simulink model "Scaler"  (Simulink 7.0)
settings: Solver=ode45  StartTime=0.0  StopTime=10.0  RelTol=1e-3
settings Model: Creator=volgy  LastModifiedBy=volgy

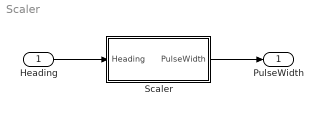
== system Scaler ==
  Heading : Inport  OutDataType=sfix(16)  OutScaling=2^0
  Scaler : Subsystem
  PulseWidth : Outport  OutDataType=sfix(16)  OutScaling=2^0
  wires:
  Heading/1 -> Scaler/1(Heading)
  Scaler/1(PulseWidth) -> PulseWidth/1

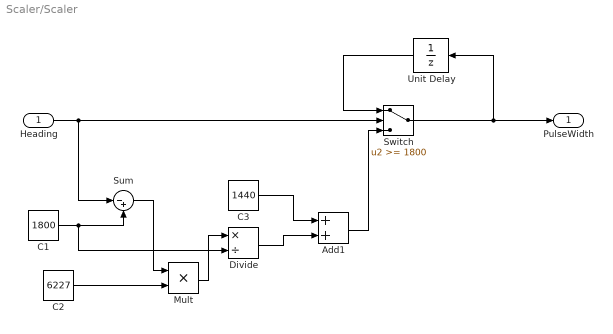
== system Scaler/Scaler ==
  Heading : Inport  OutDataType=sfix(16)  OutScaling=2^0
  Add1 : Sum  OutDataType=sfix(16)  OutScaling=2^-10
  C1 : Constant  Value=1800  OutDataType=sfix(16)  OutScaling=2^0  SampleTime=Inf
  C2 : Constant  Value=6227  OutDataType=sfix(16)  OutScaling=2^0  SampleTime=Inf
  C3 : Constant  Value=1440  OutDataType=sfix(16)  OutScaling=2^0  SampleTime=Inf
  Divide : Product  Inputs=*/  OutDataType=sfix(16)  OutScaling=2^-10
  Mult : Product  Inputs=**  OutDataType=sfix(16)  OutScaling=2^-10
  Sum : Sum  Inputs=|-+  OutDataType=sfix(16)  OutScaling=2^0
  Switch : Switch  Threshold=1800
  Unit Delay : UnitDelay  Orientation=left  X0=1440
  PulseWidth : Outport  OutDataType=sfix(16)  OutScaling=2^0
  wires:
  Unit Delay/1 -> Switch/1
  Add1/1 -> Switch/3
  Divide/1 -> Add1/2
  Mult/1 -> Divide/1
  Sum/1 -> Mult/1
  Switch/1 -> PulseWidth/1, Unit Delay/1
  C3/1 -> Add1/1
  C2/1 -> Mult/2
  C1/1 -> Sum/2, Divide/2
  Heading/1 -> Sum/1, Switch/2
